simulink model "Pacemaker_final"  (R2021b)
settings: Solver=FixedStepAuto  StartTime=0.0  StopTime=inf  FixedStep=0.001  RelTol=1e-3  EnableMultiTasking=on
model workspace (MAT data in the model file):
  parameter : Simulink.Parameter (value not decoded)
undefined symbols (not defined in the file): A0, A1, D0, D1, D10, D11, D12, D13, D2, D3, D4, D5, D6, D7, D8, D9, PTA0, PTA1, PTA2, PTB2, PTB23, PTB3, PTB9, PTC16, PTC17, PTC2, PTC3, PTC4, PTD0, PTD1, PTD2, PTD3
libraries: simulink x25, frdmk64flib x22, etargetslib x2
(part 2 of 2)

== stateflow chart Pacemaker_final/Pacing ==
  state INIT
  state AOO
  state VOO
  state AAI
  state VVI
  state DOO
  state AOOR
  state VOOR
  state AAIR
  state VVIR
  state DOOR
  (default) -> INIT
  AOO -> INIT : [MODE~=1]
  INIT -> AOO [order 5] : [MODE==1]
  VOO -> INIT : [MODE~=2]
  INIT -> VOO [order 6] : [MODE==2]
  AAI -> INIT : [MODE~=3]
  INIT -> AAI [order 2] : [MODE==3]
  VVI -> INIT : [MODE~=4]
  INIT -> VVI [order 3] : [MODE==4]
  DOO -> INIT : [MODE~=5]
  INIT -> DOO [order 7] : [MODE==5]
  AOOR -> INIT : [MODE~=6]
  INIT -> AOOR [order 8] : [MODE==6]
  VOOR -> INIT : [MODE~=7]
  INIT -> VOOR [order 1] : [MODE==7]
  AAIR -> INIT : [MODE~=8]
  INIT -> AAIR [order 9] : [MODE==8]
  VVIR -> INIT : [MODE~=9]
  INIT -> VVIR [order 10] : [MODE==9]
  DOOR -> INIT : [MODE~=10]
  INIT -> DOOR [order 4] : [MODE==10]
  data: sf_internal_action_state_placeholder_data local double size=1 =0; sf_internal_action_state_placeholder_data local double size=1 =0; sf_internal_action_state_placeholder_data local double size=1 =0; sf_internal_action_state_placeholder_data local double size=1 =0; sf_internal_action_state_placeholder_data local double size=1 =0; sf_internal_action_state_placeholder_data local double size=1 =0; sf_internal_action_state_placeholder_data local double size=1 =0; sf_internal_action_state_placeholder_data local double size=1 =0; sf_internal_action_state_placeholder_data local double size=1 =0; sf_internal_action_state_placeholder_data local double size=1 =0; ATR_CMP_DETECT input; VENT_CMP_DETECT input; Accel input double; MODE input uint8; ATR_AMP input double; Pulse_Width_atrium input uint16; LRL input double; ATR_PACE_CTRL output boolean; VENT_PACE_CTRL output boolean; PACING_REF_PWM output uint8; PACE_CHARGE_CTRL output boolean; ATR_GND_CTRL output boolean; Z_ATR_CTRL output boolean; Z_VENT_CTRL output boolean; VENT_GND_CTRL output boolean; PACE_GND_CTRL output boolean; APR input uint16; VRP input uint16; Pulse_Width_ventricle input uint16; AV_DEALAY input uint16; reaction input; recovery input; threshold input; MSR input; VENT_AMP input double

== stateflow chart Pacemaker_final/Pacing/VVI/Chart ==
  state Charging_and_Discharging
    entry:
    PACE_GND_CTRL=true;
    ATR_PACE_CTRL=false;
    VENT_PACE_CTRL=false;
    PACING_REF_PWM=uint8(Amplitude*20);
    PACE_CHARGE_CTRL=true;
    Z_ATR_CTRL=false;
    Z_VENT_CTRL=false;
    ATR_GND_CTRL=false;
    VENT_GND_CTRL=true;
  state V_Pacing
    entry:
    PACE_CHARGE_CTRL=false;
    PACE_GND_CTRL=true;
    ATR_GND_CTRL=false;
    Z_ATR_CTRL=false;
    Z_VENT_CTRL=false;
    VENT_GND_CTRL=false;
    ATR_PACE_CTRL=false;
    VENT_PACE_CTRL=true;
    PACED=true;
  (junction 69) -> Charging_and_Discharging [order 1] : [SENSED==true]{PACED=false}
  (default) -> Charging_and_Discharging
  Charging_and_Discharging -> (junction 69) [order 2] : after(VRP, msec)[PACED==false]
  (junction 69) -> V_Pacing [order 2] : after(LRL-VRP, msec)
  (junction 70) -> V_Pacing [order 2] : after(LRL-VRP, msec)
  Charging_and_Discharging -> (junction 70) [order 1] : after(VRP-PULSE_WIDTH, msec)[PACED==true]
  (junction 70) -> Charging_and_Discharging [order 1] : [SENSED==true]{PACED=false}
  V_Pacing -> Charging_and_Discharging : after(PULSE_WIDTH, msec)
  data: SENSED input boolean; VRP input uint16; ATR_PACE_CTRL output boolean; VENT_PACE_CTRL output boolean; PACING_REF_PWM output uint8; Amplitude input double; PACE_CHARGE_CTRL output boolean; ATR_GND_CTRL output boolean; Z_ATR_CTRL output boolean; Z_VENT_CTRL output boolean; VENT_GND_CTRL output boolean; PACE_GND_CTRL output boolean; PULSE_WIDTH input uint16; LRL input uint16; PACED local boolean =false

== stateflow chart Pacemaker_final/Pacing/DOO/Chart ==
  state A_Charging
    entry:
    PACE_GND_CTRL=true;
    ATR_PACE_CTRL=false;
    VENT_PACE_CTRL=false;
    PACING_REF_PWM=uint8(A_Amplitude*20);
    PACE_CHARGE_CTRL=true;
    Z_ATR_CTRL=false;
    Z_VENT_CTRL=false;
    VENT_GND_CTRL=true;
    ATR_GND_CTRL=false;
  state A_Pacing
    entry:
    PACE_CHARGE_CTRL=false;
    PACE_GND_CTRL=true;
    ATR_GND_CTRL=false;
    Z_ATR_CTRL=false;
    Z_VENT_CTRL=false;
    VENT_GND_CTRL=false;
    VENT_PACE_CTRL=false;
    ATR_PACE_CTRL=true;
  state V_Pacing
    entry:
    PACE_CHARGE_CTRL=false;
    PACE_GND_CTRL=true;
    ATR_GND_CTRL=false;
    Z_ATR_CTRL=false;
    Z_VENT_CTRL=false;
    VENT_GND_CTRL=false;
    VENT_PACE_CTRL=true;
    ATR_PACE_CTRL=false;
  state V_Charging
    entry:
    PACE_GND_CTRL=true;
    ATR_PACE_CTRL=false;
    VENT_PACE_CTRL=false;
    PACING_REF_PWM=uint8(V_Amplitude*20);
    PACE_CHARGE_CTRL=true;
    Z_ATR_CTRL=false;
    Z_VENT_CTRL=false;
    VENT_GND_CTRL=false;
    ATR_GND_CTRL=true;
  (default) -> A_Charging
  A_Charging -> A_Pacing : after(INTERVAL-VENT_PULSE_WIDTH-AV_DELAY, msec)
  A_Pacing -> V_Charging : after(ATR_PULSE_WIDTH,msec)
  V_Pacing -> A_Charging : after(VENT_PULSE_WIDTH,msec)
  V_Charging -> V_Pacing : after(AV_DELAY-ATR_PULSE_WIDTH,msec)
  data: ATR_PACE_CTRL output boolean; VENT_PACE_CTRL output boolean; PACING_REF_PWM output uint8; V_Amplitude input double; PACE_CHARGE_CTRL output boolean; ATR_GND_CTRL output boolean; Z_ATR_CTRL output boolean; Z_VENT_CTRL output boolean; VENT_GND_CTRL output boolean; PACE_GND_CTRL output boolean; VENT_PULSE_WIDTH input uint16; ATR_PULSE_WIDTH input uint16; INTERVAL input uint16; AV_DELAY input uint16; A_Amplitude input double

== stateflow chart Pacemaker_final/Pacing/AOOR/Chart ==
  state Charging_and_Discharging
    entry:
    PACE_GND_CTRL=true;
    ATR_PACE_CTRL=false;
    VENT_PACE_CTRL=false;
    PACING_REF_PWM=uint8(Amplitude*20);
    PACE_CHARGE_CTRL=true;
    Z_ATR_CTRL=false;
    Z_VENT_CTRL=false;
    VENT_GND_CTRL=false;
    ATR_GND_CTRL=true;
  state A_Pacing
    entry:
    PACE_CHARGE_CTRL=false;
    PACE_GND_CTRL=true;
    ATR_GND_CTRL=false;
    Z_ATR_CTRL=false;
    Z_VENT_CTRL=false;
    VENT_GND_CTRL=false;
    VENT_PACE_CTRL=false;
    ATR_PACE_CTRL=true;
  (default) -> Charging_and_Discharging
  Charging_and_Discharging -> A_Pacing : after(LRL-PULSE_WIDTH, msec)
  A_Pacing -> Charging_and_Discharging : after(PULSE_WIDTH, msec)
  data: ATR_PACE_CTRL output boolean; VENT_PACE_CTRL output boolean; PACING_REF_PWM output uint8; Amplitude input double; PACE_CHARGE_CTRL output boolean; ATR_GND_CTRL output boolean; Z_ATR_CTRL output boolean; Z_VENT_CTRL output boolean; VENT_GND_CTRL output boolean; PACE_GND_CTRL output boolean; PULSE_WIDTH input uint16; LRL input uint16

== stateflow chart Pacemaker_final/Pacing/AOOR/rate adaptive ==
  state start
    entry:
    OUTPUT_PACE = LRL;
  state IDLE
  state increase_pace
    entry:
    OUTPUT_PACE = OUTPUT_PACE + increment;
  state calculate_increment
    entry:
    increment = 2.5*(TARGET_RATE-OUTPUT_PACE) / REACTION_TIME;
  state calculate_decrement
    entry:
    decrement = (OUTPUT_PACE - TARGET_RATE) / RECOVERY_TIME;
  state decrease_pace
    entry:
    OUTPUT_PACE = OUTPUT_PACE - decrement;
  (default) -> start
  increase_pace -> IDLE [order 1] : [OUTPUT_PACE == TARGET_RATE]
  start -> IDLE
  calculate_increment -> increase_pace
  decrease_pace -> IDLE : after(500,msec)
  IDLE -> calculate_increment [order 1] : [TARGET_RATE > OUTPUT_PACE]
  IDLE -> calculate_decrement [order 2] : [TARGET_RATE < OUTPUT_PACE]
  increase_pace -> calculate_decrement [order 3] : [TARGET_RATE < OUTPUT_PACE]
  increase_pace -> increase_pace [order 2] : after(1,sec)
  calculate_decrement -> decrease_pace
  data: MSR input double; LRL input double; REACTION_TIME input double; RECOVERY_TIME input double; ACTIVITY_THRESHOLD input single; OUTPUT_PACE output double; TARGET_RATE input double; decrement local double; increment local double

== stateflow chart Pacemaker_final/Pacing/VOOR/Chart ==
  state Charging_and_Discharging
    entry:
    PACE_GND_CTRL=true;
    ATR_PACE_CTRL=false;
    VENT_PACE_CTRL=false;
    PACING_REF_PWM=uint8(Amplitude*20);
    PACE_CHARGE_CTRL=true;
    Z_ATR_CTRL=false;
    Z_VENT_CTRL=false;
    ATR_GND_CTRL=false;
    VENT_GND_CTRL=true;
  state V_Pacing
    entry:
    PACE_CHARGE_CTRL=false;
    PACE_GND_CTRL=true;
    ATR_GND_CTRL=false;
    Z_ATR_CTRL=false;
    Z_VENT_CTRL=false;
    VENT_GND_CTRL=false;
    ATR_PACE_CTRL=false;
    VENT_PACE_CTRL=true;
  (default) -> Charging_and_Discharging
  Charging_and_Discharging -> V_Pacing : after(LRL-PULSE_WIDTH, msec)
  V_Pacing -> Charging_and_Discharging : after(PULSE_WIDTH, msec)
  data: ATR_PACE_CTRL output boolean; VENT_PACE_CTRL output boolean; PACING_REF_PWM output uint8; Amplitude input double; PACE_CHARGE_CTRL output boolean; ATR_GND_CTRL output boolean; Z_ATR_CTRL output boolean; Z_VENT_CTRL output boolean; VENT_GND_CTRL output boolean; PACE_GND_CTRL output boolean; PULSE_WIDTH input uint16; LRL input uint16

== stateflow chart Pacemaker_final/Pacing/AAIR/Chart1 ==
  state Charging_and_Discharging
    entry:
    PACE_GND_CTRL=true;
    ATR_PACE_CTRL=false;
    VENT_PACE_CTRL=false;
    PACING_REF_PWM=uint8(Amplitude*20);
    PACE_CHARGE_CTRL=true;
    Z_ATR_CTRL=false;
    Z_VENT_CTRL=false;
    VENT_GND_CTRL=false;
    ATR_GND_CTRL=true;
  state A_Pacing
    entry:
    PACE_CHARGE_CTRL=false;
    PACE_GND_CTRL=true;
    ATR_GND_CTRL=false;
    Z_ATR_CTRL=false;
    Z_VENT_CTRL=false;
    VENT_GND_CTRL=false;
    VENT_PACE_CTRL=false;
    ATR_PACE_CTRL=true;
    PACED=true;
  (junction 65) -> Charging_and_Discharging [order 2] : [SENSED==true]{PACED=false}
  Charging_and_Discharging -> (junction 65) [order 1] : after(ARP, msec)[PACED==false]
  (junction 65) -> A_Pacing [order 1] : after(LRL-ARP, msec)
  (default) -> Charging_and_Discharging
  Charging_and_Discharging -> (junction 62) [order 2] : after(ARP-PULSE_WIDTH, msec)[PACED==true]
  (junction 62) -> A_Pacing [order 1] : after(LRL-ARP, msec)
  (junction 62) -> Charging_and_Discharging [order 2] : [SENSED==true]{PACED=false}
  A_Pacing -> Charging_and_Discharging : after(PULSE_WIDTH, msec)
  data: SENSED input boolean; ARP input uint16; ATR_PACE_CTRL output boolean; VENT_PACE_CTRL output boolean; PACING_REF_PWM output uint8; Amplitude input double; PACE_CHARGE_CTRL output boolean; ATR_GND_CTRL output boolean; Z_ATR_CTRL output boolean; Z_VENT_CTRL output boolean; VENT_GND_CTRL output boolean; PACE_GND_CTRL output boolean; PULSE_WIDTH input uint16; LRL input uint16; PACED local boolean =false

== stateflow chart Pacemaker_final/Pacing/VVIR/Chart ==
  state Charging_and_Discharging
    entry:
    PACE_GND_CTRL=true;
    ATR_PACE_CTRL=false;
    VENT_PACE_CTRL=false;
    PACING_REF_PWM=uint8(Amplitude*20);
    PACE_CHARGE_CTRL=true;
    Z_ATR_CTRL=false;
    Z_VENT_CTRL=false;
    ATR_GND_CTRL=false;
    VENT_GND_CTRL=true;
  state V_Pacing
    entry:
    PACE_CHARGE_CTRL=false;
    PACE_GND_CTRL=true;
    ATR_GND_CTRL=false;
    Z_ATR_CTRL=false;
    Z_VENT_CTRL=false;
    VENT_GND_CTRL=false;
    ATR_PACE_CTRL=false;
    VENT_PACE_CTRL=true;
    PACED=true;
  (junction 69) -> Charging_and_Discharging [order 1] : [SENSED==true]{PACED=false}
  (default) -> Charging_and_Discharging
  Charging_and_Discharging -> (junction 69) [order 2] : after(VRP, msec)[PACED==false]
  (junction 69) -> V_Pacing [order 2] : after(LRL-VRP, msec)
  (junction 70) -> V_Pacing [order 2] : after(LRL-VRP, msec)
  Charging_and_Discharging -> (junction 70) [order 1] : after(VRP-PULSE_WIDTH, msec)[PACED==true]
  (junction 70) -> Charging_and_Discharging [order 1] : [SENSED==true]{PACED=false}
  V_Pacing -> Charging_and_Discharging : after(PULSE_WIDTH, msec)
  data: SENSED input boolean; VRP input uint16; ATR_PACE_CTRL output boolean; VENT_PACE_CTRL output boolean; PACING_REF_PWM output uint8; Amplitude input double; PACE_CHARGE_CTRL output boolean; ATR_GND_CTRL output boolean; Z_ATR_CTRL output boolean; Z_VENT_CTRL output boolean; VENT_GND_CTRL output boolean; PACE_GND_CTRL output boolean; PULSE_WIDTH input uint16; LRL input uint16; PACED local boolean =false

== stateflow chart Pacemaker_final/Pacing/DOOR/Pacing ==
  state A_Charging
    entry:
    PACE_GND_CTRL=true;
    ATR_PACE_CTRL=false;
    VENT_PACE_CTRL=false;
    PACING_REF_PWM=uint8(A_Amplitude*20);
    PACE_CHARGE_CTRL=true;
    Z_ATR_CTRL=false;
    Z_VENT_CTRL=false;
    VENT_GND_CTRL=true;
    ATR_GND_CTRL=false;
  state A_Pacing
    entry:
    PACE_CHARGE_CTRL=false;
    PACE_GND_CTRL=true;
    ATR_GND_CTRL=false;
    Z_ATR_CTRL=false;
    Z_VENT_CTRL=false;
    VENT_GND_CTRL=false;
    VENT_PACE_CTRL=false;
    ATR_PACE_CTRL=true;
  state V_Pacing
    entry:
    PACE_CHARGE_CTRL=false;
    PACE_GND_CTRL=true;
    ATR_GND_CTRL=false;
    Z_ATR_CTRL=false;
    Z_VENT_CTRL=false;
    VENT_GND_CTRL=false;
    VENT_PACE_CTRL=true;
    ATR_PACE_CTRL=false;
  state V_Charging
    entry:
    PACE_GND_CTRL=true;
    ATR_PACE_CTRL=false;
    VENT_PACE_CTRL=false;
    PACING_REF_PWM=uint8(V_Amplitude*20);
    PACE_CHARGE_CTRL=true;
    Z_ATR_CTRL=false;
    Z_VENT_CTRL=false;
    VENT_GND_CTRL=false;
    ATR_GND_CTRL=true;
  (default) -> A_Charging
  A_Charging -> A_Pacing : after(INTERVAL-VENT_PULSE_WIDTH-AV_DELAY, msec)
  A_Pacing -> V_Charging : after(ATR_PULSE_WIDTH,msec)
  V_Pacing -> A_Charging : after(VENT_PULSE_WIDTH,msec)
  V_Charging -> V_Pacing : after(AV_DELAY-ATR_PULSE_WIDTH,msec)
  data: ATR_PACE_CTRL output boolean; VENT_PACE_CTRL output boolean; PACING_REF_PWM output uint8; A_Amplitude input double; PACE_CHARGE_CTRL output boolean; ATR_GND_CTRL output boolean; Z_ATR_CTRL output boolean; Z_VENT_CTRL output boolean; VENT_GND_CTRL output boolean; PACE_GND_CTRL output boolean; VENT_PULSE_WIDTH input uint16; ATR_PULSE_WIDTH input uint16; INTERVAL input uint16; AV_DELAY input uint16; V_Amplitude input double

== stateflow chart Pacemaker_final/Pacing/AAI/Chart1 ==
  state Charging_and_Discharging
    entry:
    PACE_GND_CTRL=true;
    ATR_PACE_CTRL=false;
    VENT_PACE_CTRL=false;
    PACING_REF_PWM=uint8(Amplitude*20);
    PACE_CHARGE_CTRL=true;
    Z_ATR_CTRL=false;
    Z_VENT_CTRL=false;
    VENT_GND_CTRL=false;
    ATR_GND_CTRL=true;
  state A_Pacing
    entry:
    PACE_CHARGE_CTRL=false;
    PACE_GND_CTRL=true;
    ATR_GND_CTRL=false;
    Z_ATR_CTRL=false;
    Z_VENT_CTRL=false;
    VENT_GND_CTRL=false;
    VENT_PACE_CTRL=false;
    ATR_PACE_CTRL=true;
    PACED=true;
  (junction 65) -> Charging_and_Discharging [order 2] : [SENSED==true]{PACED=false}
  Charging_and_Discharging -> (junction 65) [order 1] : after(ARP, msec)[PACED==false]
  (junction 65) -> A_Pacing [order 1] : after(LRL-ARP, msec)
  (default) -> Charging_and_Discharging
  Charging_and_Discharging -> (junction 62) [order 2] : after(ARP-PULSE_WIDTH, msec)[PACED==true]
  (junction 62) -> A_Pacing [order 1] : after(LRL-ARP, msec)
  (junction 62) -> Charging_and_Discharging [order 2] : [SENSED==true]{PACED=false}
  A_Pacing -> Charging_and_Discharging : after(PULSE_WIDTH, msec)
  data: SENSED input boolean; ARP input uint16; ATR_PACE_CTRL output boolean; VENT_PACE_CTRL output boolean; PACING_REF_PWM output uint8; Amplitude input double; PACE_CHARGE_CTRL output boolean; ATR_GND_CTRL output boolean; Z_ATR_CTRL output boolean; Z_VENT_CTRL output boolean; VENT_GND_CTRL output boolean; PACE_GND_CTRL output boolean; PULSE_WIDTH input uint16; LRL input uint16; PACED local boolean =false

== stateflow chart Pacemaker_final/Pacing/VOOR/rate adaptive ==
  state start
    entry:
    OUTPUT_PACE = LRL;
  state IDLE
  state increase_pace
    entry:
    OUTPUT_PACE = OUTPUT_PACE + increment;
  state calculate_increment
    entry:
    increment = 2.5*(TARGET_RATE-OUTPUT_PACE) / REACTION_TIME;
  state calculate_decrement
    entry:
    decrement = (OUTPUT_PACE - TARGET_RATE) / RECOVERY_TIME;
  state decrease_pace
    entry:
    OUTPUT_PACE = OUTPUT_PACE - decrement;
  (default) -> start
  increase_pace -> IDLE [order 1] : [OUTPUT_PACE == TARGET_RATE]
  start -> IDLE
  calculate_increment -> increase_pace
  decrease_pace -> IDLE : after(500,msec)
  IDLE -> calculate_increment [order 1] : [TARGET_RATE > OUTPUT_PACE]
  IDLE -> calculate_decrement [order 2] : [TARGET_RATE < OUTPUT_PACE]
  increase_pace -> calculate_decrement [order 3] : [TARGET_RATE < OUTPUT_PACE]
  increase_pace -> increase_pace [order 2] : after(1,sec)
  calculate_decrement -> decrease_pace
  data: MSR input double; LRL input double; REACTION_TIME input double; RECOVERY_TIME input double; ACTIVITY_THRESHOLD input single; OUTPUT_PACE output double; TARGET_RATE input double; decrement local double; increment local double

== stateflow chart Pacemaker_final/Pacing/AAIR/rate adaptive ==
  state start
    entry:
    OUTPUT_PACE = LRL;
  state IDLE
  state increase_pace
    entry:
    OUTPUT_PACE = OUTPUT_PACE + increment;
  state calculate_increment
    entry:
    increment = 2.5*(TARGET_RATE-OUTPUT_PACE) / REACTION_TIME;
  state calculate_decrement
    entry:
    decrement = (OUTPUT_PACE - TARGET_RATE) / RECOVERY_TIME;
  state decrease_pace
    entry:
    OUTPUT_PACE = OUTPUT_PACE - decrement;
  (default) -> start
  increase_pace -> IDLE [order 1] : [OUTPUT_PACE == TARGET_RATE]
  start -> IDLE
  calculate_increment -> increase_pace
  decrease_pace -> IDLE : after(500,msec)
  IDLE -> calculate_increment [order 1] : [TARGET_RATE > OUTPUT_PACE]
  IDLE -> calculate_decrement [order 2] : [TARGET_RATE < OUTPUT_PACE]
  increase_pace -> calculate_decrement [order 3] : [TARGET_RATE < OUTPUT_PACE]
  increase_pace -> increase_pace [order 2] : after(1,sec)
  calculate_decrement -> decrease_pace
  data: MSR input double; LRL input double; REACTION_TIME input double; RECOVERY_TIME input double; ACTIVITY_THRESHOLD input single; OUTPUT_PACE output double; TARGET_RATE input double; decrement local double; increment local double

== stateflow chart Pacemaker_final/Pacing/VVIR/rate adaptive ==
  state start
    entry:
    OUTPUT_PACE = LRL;
  state IDLE
  state increase_pace
    entry:
    OUTPUT_PACE = OUTPUT_PACE + increment;
  state calculate_increment
    entry:
    increment = 2.5*(TARGET_RATE-OUTPUT_PACE) / REACTION_TIME;
  state calculate_decrement
    entry:
    decrement = (OUTPUT_PACE - TARGET_RATE) / RECOVERY_TIME;
  state decrease_pace
    entry:
    OUTPUT_PACE = OUTPUT_PACE - decrement;
  (default) -> start
  increase_pace -> IDLE [order 1] : [OUTPUT_PACE == TARGET_RATE]
  start -> IDLE
  calculate_increment -> increase_pace
  decrease_pace -> IDLE : after(500,msec)
  IDLE -> calculate_increment [order 1] : [TARGET_RATE > OUTPUT_PACE]
  IDLE -> calculate_decrement [order 2] : [TARGET_RATE < OUTPUT_PACE]
  increase_pace -> calculate_decrement [order 3] : [TARGET_RATE < OUTPUT_PACE]
  increase_pace -> increase_pace [order 2] : after(1,sec)
  calculate_decrement -> decrease_pace
  data: MSR input double; LRL input double; REACTION_TIME input double; RECOVERY_TIME input double; ACTIVITY_THRESHOLD input single; OUTPUT_PACE output double; TARGET_RATE input double; decrement local double; increment local double

== stateflow chart Pacemaker_final/Pacing/DOOR/rate adaptive ==
  state start
    entry:
    OUTPUT_PACE = LRL;
  state IDLE
  state increase_pace
    entry:
    OUTPUT_PACE = OUTPUT_PACE + increment;
  state calculate_increment
    entry:
    increment = 2.5*(TARGET_RATE-OUTPUT_PACE) / REACTION_TIME;
  state calculate_decrement
    entry:
    decrement = (OUTPUT_PACE - TARGET_RATE) / RECOVERY_TIME;
  state decrease_pace
    entry:
    OUTPUT_PACE = OUTPUT_PACE - decrement;
  (default) -> start
  increase_pace -> IDLE [order 1] : [OUTPUT_PACE == TARGET_RATE]
  start -> IDLE
  calculate_increment -> increase_pace
  decrease_pace -> IDLE : after(500,msec)
  IDLE -> calculate_increment [order 1] : [TARGET_RATE > OUTPUT_PACE]
  IDLE -> calculate_decrement [order 2] : [TARGET_RATE < OUTPUT_PACE]
  increase_pace -> calculate_decrement [order 3] : [TARGET_RATE < OUTPUT_PACE]
  increase_pace -> increase_pace [order 2] : after(1,sec)
  calculate_decrement -> decrease_pace
  data: MSR input double; LRL input double; REACTION_TIME input double; RECOVERY_TIME input double; ACTIVITY_THRESHOLD input single; OUTPUT_PACE output double; TARGET_RATE input double; decrement local double; increment local double

== stateflow chart Pacemaker_final/Serial communication ==
  state SET_PARAMETERS
    entry:
    confirm=1;
    Mode = rxdata(2);
    ATR_AMP = typecast(rxdata(3:10), 'double');
    Pulse_width_atrium = typecast(rxdata(11:12), 'uint16');
    ARP = typecast(rxdata(13:14), 'uint16');
    VRP = typecast(rxdata(15:16), 'uint16');
    VENT_AMP = typecast(rxdata(17:24), 'double');
    Pulse_width_ventricle =typecast(rxdata(25:26), 'uint16');
    AV_DELAY = typecast(rxdata(27:28), 'uint16');
    reaction = typecast(rxdata(29:36), 'double');
    recovery = typecast(rxdata(37:44), 'double');
    threshold = typecast(rxdata(45:48), 'single');
    MSR=typecast(rxdata(49:56), 'double');
    LRL = typecast(rxdata(57:58), 'uint16');
  state start
    entry:
    Mode = 1;
    LRL = 120;
    VENT_AMP = 4;
    Pulse_width_ventricle = 1;
    ATR_AMP = 4;
    Pulse_width_atrium = 1;
    ARP = 200;
    VRP = 200;
    threshold = 1;
    reaction = 15;
    recovery = 15;
    AV_DELAY = 150;
    MSR=160;
  state IDLE
    entry:
    confirm=0;
    red=true;
  state egram_and_confimation
  (default) -> start
  (junction 36) -> IDLE [order 2]
  (junction 38) -> SET_PARAMETERS [order 1] : [rxdata(59)==hex2dec('17')]{red=false}
  start -> IDLE
  IDLE -> (junction 36) : [status==0]{blue=true}
  (junction 36) -> (junction 38) [order 1] : [rxdata(1)==hex2dec('16')]{green=true}
  (junction 38) -> egram_and_confimation [order 2] : [rxdata(2)==hex2dec('26')]
  egram_and_confimation -> IDLE [order 1] : [confirm==1]{green=false}
  (junction 46) -> IDLE [order 1] : [rxdata(1)==2]{green=false}
  SET_PARAMETERS -> egram_and_confimation : {blue= false}
  egram_and_confimation -> (junction 46) [order 2] : [status==0]
  (junction 46) -> egram_and_confimation [order 2]
  data: sf_internal_action_state_placeholder_data local double size=1 =0; Mode output uint8; reaction output double; VENT_AMP output double; threshold output single; MSR output double; recovery output double; ATR_AMP output double; LRL output uint16; VRP output uint16; rxdata input uint8; status input uint8; confirm local uint8; ARP output uint16; AV_DELAY output uint16; Pulse_width_atrium output uint16; Pulse_width_ventricle output uint16; red output boolean =false; blue output boolean =false; green output boolean =false

== stateflow chart Pacemaker_final/Pacing/AOO/Chart ==
  state Charging_and_Discharging
    entry:
    PACE_GND_CTRL=true;
    ATR_PACE_CTRL=false;
    VENT_PACE_CTRL=false;
    PACING_REF_PWM=uint8(Amplitude*20);
    PACE_CHARGE_CTRL=true;
    Z_ATR_CTRL=false;
    Z_VENT_CTRL=false;
    VENT_GND_CTRL=false;
    ATR_GND_CTRL=true;
  state A_Pacing
    entry:
    PACE_CHARGE_CTRL=false;
    PACE_GND_CTRL=true;
    ATR_GND_CTRL=false;
    Z_ATR_CTRL=false;
    Z_VENT_CTRL=false;
    VENT_GND_CTRL=false;
    VENT_PACE_CTRL=false;
    ATR_PACE_CTRL=true;
  (default) -> Charging_and_Discharging
  Charging_and_Discharging -> A_Pacing : after(LRL-PULSE_WIDTH, msec)
  A_Pacing -> Charging_and_Discharging : after(PULSE_WIDTH, msec)
  data: ATR_PACE_CTRL output boolean; VENT_PACE_CTRL output boolean; PACING_REF_PWM output uint8; Amplitude input double; PACE_CHARGE_CTRL output boolean; ATR_GND_CTRL output boolean; Z_ATR_CTRL output boolean; Z_VENT_CTRL output boolean; VENT_GND_CTRL output boolean; PACE_GND_CTRL output boolean; PULSE_WIDTH input uint16; LRL input uint16
